simulink model "MPCstatespace"  (R2023b)
settings: Solver=FixedStepAuto  StartTime=0.0  StopTime=10.0  FixedStep=0.05  RelTol=1e-3
undefined symbols (not defined in the file): A, B, C, D, DiscIntNeverNeededParam
libraries: mpclib x1
settings Model: Creator=lxy18  LastModifiedBy=lxy18

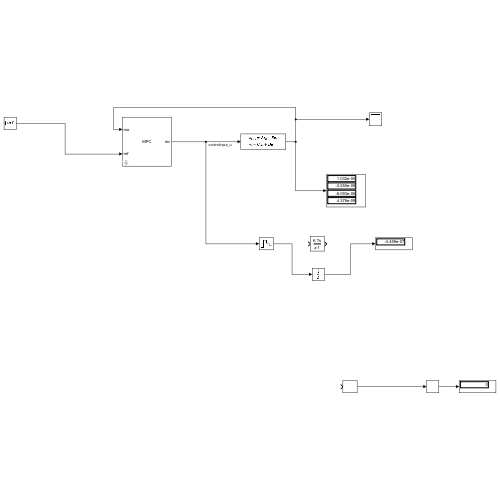
[thumbnail: Simulink's stored preview of the top-level diagram]
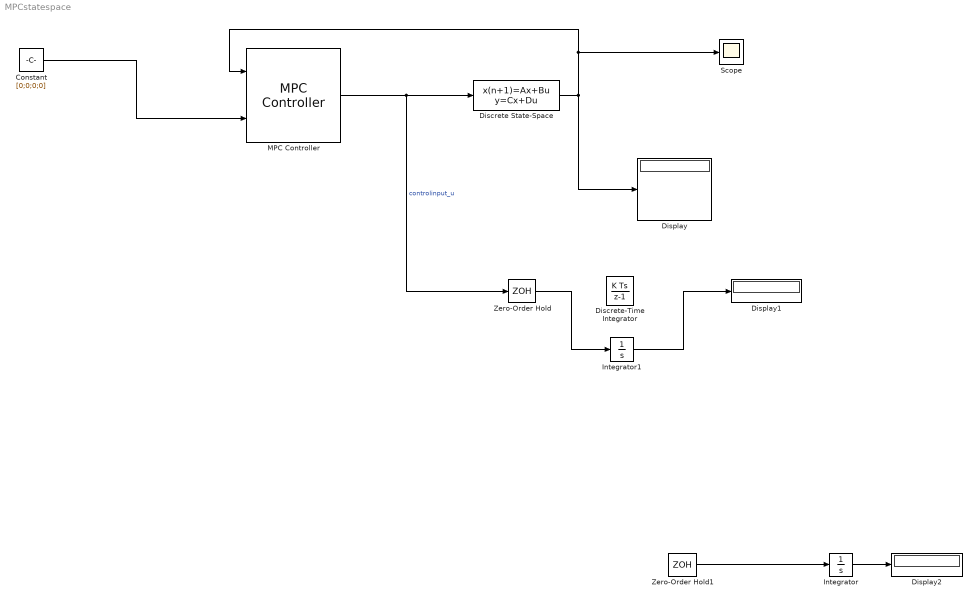
== system MPCstatespace ==
  Constant : Constant  Value=[0;0;0;0]  SampleTime=0.05
  Discrete State-Space : DiscreteStateSpace  A=A  B=B  C=C  D=D  InitialCondition=[ pi / 180;pi / 180;0;0]  SampleTime=0.05
  Discrete-Time Integrator : DiscreteIntegrator  SampleTime=-1  ICPrevOutput=DiscIntNeverNeededParam  ICPrevScaledInput=DiscIntNeverNeededParam
  Display : Display
  Display1 : Display
  Display2 : Display
  Integrator : Integrator
  Integrator1 : Integrator
  MPC Controller : mpclib/MPC Controller  SCDEnableBlockLinearizationSpecification=on  mpcobj=mpc_obj  is_multiple=0  enable_value=0  return_u0=off  updateMPCinCallerWorkspace=on  md_inport=off  mv_inport=off  uref_inport=off  return_cost=off  return_mvseq=off  return_qpstatus=off  return_xseq=off  return_state=off  return_ovseq=off  state_inport=off  umin_inport=off  umax_inport=off  ymin_inport=off  ymax_inport=off  cc_inport=off  ywt_inport=off  uwt_inport=off  duwt_inport=off  rhoeps_inport=off  pm_inport=off  MaximumP=10  HorizonChoice=FixedHorizon  n_ts=0.05  n_p=20  n_mv=1  n_md=0  n_ud=0  n_mo=4  n_uo=0  BlockDataType=double  SampleTimeInherited=off  switch_inport=off
  Scope : Scope
  Zero-Order Hold : ZeroOrderHold  SampleTime=-1
  Zero-Order Hold1 : ZeroOrderHold  SampleTime=-1
  wires:
  MPC Controller/1 -> Zero-Order Hold/1, Discrete State-Space/1  "controlinput_u"
  Discrete State-Space/1 -> Scope/1, MPC Controller/1, Display/1
  Constant/1 -> MPC Controller/2
  Zero-Order Hold1/1 -> Integrator/1
  Integrator/1 -> Display2/1
  Zero-Order Hold/1 -> Integrator1/1
  Integrator1/1 -> Display1/1
